simulink subsystem "PvtSubSys_LATC"  (R2020b)
settings: Solver=VariableStepAuto  StartTime=0.0  StopTime=10.0  RelTol=1e-3
values from neighbouring files (symbols this model uses):
  P_Global_CharSpd_ms : value not decoded    [PubParsGlobal.sldd]
  P_Global_SteeringAngleRatio : value not decoded    [PubParsGlobal.sldd]
  P_Global_WheelBase_m : value not decoded    [PubParsGlobal.sldd]
  P_LCS_A0_Limit = 0.25    [LATC.sldd]    (also in LCS_v05.sldd)
  P_LCS_A1_Limit = 0.002    [LATC.sldd]    (also in LCS_v05.sldd)
  P_LCS_communicationTest = 1.0    [LATC.sldd]    (also in LCS_v05.sldd)
  P_LCS_Current_Offset_Test_SW = 0.0    [LATC.sldd]
  P_LCS_Current_Offset_Test_Value = 0.0    [LATC.sldd]
  P_LCS_Curvature_bp : value not decoded    [LATC.sldd]
  P_LCS_CycleTime = 0.4 0.4 0.4 0.4 0.4 0.4 0.4 0.4 0.4 0.6 0.6 0.6 0.6 0.6 0.6 0.6 0.4 0.4 0.4 0.4 0.4 0.4 0.4 0.4 0.4 0.6 0.6 0.6 0.6 0.6 0.6 0.6 0.4 0.4 0.4 0.4 0.4 0.4 0.4 0.4 0.4 0.6 0.6 0.6 0.6 0.6 0.6 0.6 0.4 0.4 0.4 0.4 0.4 0.4 0.4 0.4 0.4 0.6 0.6 0.6 0.6 0.6 0.6 0.6 0.4 0.4 0.4 0.4 0.4 0.4 0.4 0.4 0.4 0.6 0.6 0.6 0.6 0.6 0.6 0.6 0.4 0.4 0.4 0.4 0.4 0.4 0.4 0.4 0.4 0.6 0.6 0.6 0.6 0.6 0.6 0.6 0.4 0.4 0.4 0.4    [LATC.sldd]
  P_LCS_ESS_AngleSlope_Limit = 2.9    [LATC.sldd]    (also in LCS_v05.sldd)
  P_LCS_IN_Offset_Test_SW = 0.0    [LATC.sldd]    (also in LCS_v05.sldd)
  P_LCS_IN_Offset_Test_Value = 0.0    [LATC.sldd]    (also in LCS_v05.sldd)
  P_LCS_LATC_CurOffsetVehicleSpdLimitValue_degs = 7.0    [LATC.sldd]
  P_LCS_LATC_Du_Max = 20.0    [LATC.sldd]
  P_LCS_LATC_ELKAngleSlope_ratio : value not decoded    [LATC.sldd]
  P_LCS_LATC_ELKMaxLatAcc_ms2 : value not decoded    [LATC.sldd]
  P_LCS_LATC_ESSAngleSlope_ratio : value not decoded    [LATC.sldd]
  P_LCS_LATC_ESSMaxLatAcc_ms2 : value not decoded    [LATC.sldd]
  P_LCS_LATC_LCAngleSlope_ratio : value not decoded    [LATC.sldd]
  P_LCS_LATC_LCCancleMaxLatAcc_ms2 : value not decoded    [LATC.sldd]
  P_LCS_LATC_LCEcoAngleSlope_ratio : value not decoded    [LATC.sldd]
  P_LCS_LATC_LCEcoMaxLatAcc_ms2 : value not decoded    [LATC.sldd]
  P_LCS_LATC_LCKAngleSlope_ratio : value not decoded    [LATC.sldd]
  P_LCS_LATC_LCKIEAngleSlope_ratio : value not decoded    [LATC.sldd]
  P_LCS_LATC_LCKIEMaxLatAcc_ms2 : value not decoded    [LATC.sldd]
  P_LCS_LATC_LCKMaxLatAcc_ms2 : value not decoded    [LATC.sldd]
  P_LCS_LATC_LCNormalAngleSlope_ratio : value not decoded    [LATC.sldd]
  P_LCS_LATC_LCNormalMaxLatAcc_ms2 : value not decoded    [LATC.sldd]
  P_LCS_LATC_LCSportAngleSlope_ratio : value not decoded    [LATC.sldd]
  P_LCS_LATC_LCSportMaxLatAcc_ms2 : value not decoded    [LATC.sldd]
  P_LCS_LATC_LKAAngleSlope_ratio : value not decoded    [LATC.sldd]
  P_LCS_LATC_LKAMaxLatAcc_ms2 : value not decoded    [LATC.sldd]
  P_LCS_LATC_MatrixQ1_st = 0.8 0.8 1.2 1.4 1.4 1.4 2.0 2.2 2.2 2.2 2.2 2.2 2.2 2.2 2.2 2.2 0.8 0.8 1.2 1.4 1.4 1.4 2.0 2.2 2.2 2.2 2.2 2.2 2.2 2.2 2.2 2.2 0.8 0.8 1.2 1.4 1.4 1.4 2.0 2.2 2.2 2.2 2.2 2.2 2.2 2.2 2.2 2.2 0.8 0.8 1.2 1.4 1.4 1.4 2.0 2.2 2.2 2.2 2.2 2.2 2.2 2.2 2.2 2.2 0.8 0.8 1.2 1.4 1.4 1.4 2.0 2.2 2.2 2.2 2.2 2.2 2.2 2.2 2.2 2.2 0.8 0.8 1.2 1.4 1.4 1.4 2.0 2.2 2.2 2.2 2.2 2.2 2.2 2.2 2.2 2.2 0.8 0.8 1.2 1.4    [LATC.sldd]
  P_LCS_LATC_MatrixQ3_st = 20.0 20.0 20.0 20.0 20.0 15.0 15.0 15.0 15.0 15.0 15.0 15.0 15.0 13.0 13.0 13.0 20.0 20.0 20.0 20.0 20.0 15.0 15.0 15.0 15.0 15.0 15.0 15.0 15.0 13.0 13.0 13.0 20.0 20.0 20.0 20.0 20.0 15.0 15.0 15.0 15.0 15.0 15.0 15.0 15.0 13.0 13.0 13.0 20.0 20.0 20.0 20.0 20.0 15.0 15.0 15.0 15.0 15.0 15.0 15.0 15.0 13.0 13.0 13.0 20.0 20.0 20.0 20.0 20.0 15.0 15.0 15.0 15.0 15.0 15.0 15.0 15.0 13.0 13.0 13.0    [LATC.sldd]
  P_LCS_LATC_MatrixR_st = 10.0 10.0 10.0 10.0 10.0 10.0 10.0 15.0 15.0 15.0 15.0 15.0 15.0 15.0 15.0 15.0 10.0 10.0 10.0 10.0 10.0 10.0 10.0 15.0 15.0 15.0 15.0 15.0 15.0 15.0 15.0 15.0 10.0 10.0 10.0 10.0 10.0 10.0 10.0 15.0 15.0 15.0 15.0 15.0 15.0 15.0 15.0 15.0 10.0 10.0 10.0 10.0 10.0 10.0 10.0 15.0 15.0 15.0 15.0 15.0 15.0 15.0 15.0 15.0 10.0 10.0 10.0 10.0 10.0 10.0 10.0 15.0 15.0 15.0 15.0 15.0 15.0 15.0 15.0 15.0    [LATC.sldd]
  P_LCS_LATC_Max_LatAcc = 4.0    [LATC.sldd]
  P_LCS_LATC_Max_Phi = 15.0    [LATC.sldd]
  P_LCS_LATC_Max_y = 0.5    [LATC.sldd]
  P_LCS_LATC_MPC_SW = 0.0    [LATC.sldd]
  P_LCS_LATC_PreView_SW = 1.0    [LATC.sldd]
  P_LCS_LATC_SoftConstWeight = 1.0    [LATC.sldd]
  P_LCS_LATC_StateActivAngleSlopeLimit_ratio : value not decoded    [LATC.sldd]
  P_LCS_LATC_StateActiveFlg_TabX_st : value not decoded    [LATC.sldd]
  P_LCS_LATC_StateActiveHoldTime_TabY_st : value not decoded    [LATC.sldd]
  P_LCS_LATC_StateHoldTime_st = 250.0    [LATC.sldd]
  P_LCS_LATC_TarAngleFliterWindowSize = 5.0    [LATC.sldd]
  P_LCS_LATC_TarAngleLP_Time = 0.02    [LATC.sldd]
  P_LCS_LATC_U_Max = 90.0    [LATC.sldd]
  P_LCS_LCK_AngleSlope_Limit = 1.4    [LATC.sldd]
  P_LCS_LineVaildSW = 0.0    [LATC.sldd]
  P_LCS_Lookahead_Distance : value not decoded    [LATC.sldd]
  P_LCS_Lookahead_DistanceFac : value not decoded    [LATC.sldd]
  P_LCS_PLAN_CurvePreView_s = 0.3    [LATC.sldd]
  P_LCS_PLAN_CurvePreview_TabX_m : value not decoded    [LATC.sldd]
  P_LCS_PLAN_CurvePreViewFilterTime_s = 0.1    [LATC.sldd]
  P_LCS_PLAN_ELKAyDtLimit_Tab_ms3 = 1.0 1.0 1.0 1.0 1.0 1.0 1.0 1.0 1.0 1.0 1.0 1.0 1.0 1.0 1.0 1.0 1.0 1.0 1.0 1.0 1.0 1.0 1.0 1.0 1.0 1.0 1.0 1.0 1.0 1.0 1.0 1.0 1.0 1.0 1.0 1.0 1.0 1.0 1.0 1.0 1.0 1.0 1.0 1.0 1.0 1.0 1.0 1.0 1.0 1.0 1.0 1.0 1.0 1.0 1.0 1.0 1.0 1.0 1.0 1.0 1.0 1.0 1.0 1.0 1.0 1.0 1.0 1.0 1.0 1.0 1.0 1.0 1.0 1.0 1.0 1.0 1.0 1.0 1.0 1.0 1.0 1.0 1.0 1.0 1.0 1.0 1.0 1.0 1.0 1.0 1.0 1.0 1.0 1.0 1.0 1.0 1.0 1.0 1.0 1.0    [LATC.sldd]
  P_LCS_PLAN_ESSAyDtLimit_Tab_ms3 = 1.0 1.0 1.0 1.0 1.0 1.0 1.0 1.0 1.0 1.0 1.0 1.0 1.0 1.0 1.0 1.0 1.0 1.0 1.0 1.0 1.0 1.0 1.0 1.0 1.0 1.0 1.0 1.0 1.0 1.0 1.0 1.0 1.0 1.0 1.0 1.0 1.0 1.0 1.0 1.0 1.0 1.0 1.0 1.0 1.0 1.0 1.0 1.0 1.0 1.0 1.0 1.0 1.0 1.0 1.0 1.0 1.0 1.0 1.0 1.0 1.0 1.0 1.0 1.0 1.0 1.0 1.0 1.0 1.0 1.0 1.0 1.0 1.0 1.0 1.0 1.0 1.0 1.0 1.0 1.0 1.0 1.0 1.0 1.0 1.0 1.0 1.0 1.0 1.0 1.0 1.0 1.0 1.0 1.0 1.0 1.0 1.0 1.0 1.0 1.0    [LATC.sldd]
  P_LCS_PLAN_LCCancleAyDtLimit_Tab_ms3 = 1.0 1.0 1.0 1.0 1.0 1.0 1.0 1.0 1.0 1.0 1.0 1.0 1.0 1.0 1.0 1.0 1.0 1.0 1.0 1.0 1.0 1.0 1.0 1.0 1.0 1.0 1.0 1.0 1.0 1.0 1.0 1.0 1.0 1.0 1.0 1.0 1.0 1.0 1.0 1.0 1.0 1.0 1.0 1.0 1.0 1.0 1.0 1.0 1.0 1.0 1.0 1.0 1.0 1.0 1.0 1.0 1.0 1.0 1.0 1.0 1.0 1.0 1.0 1.0 1.0 1.0 1.0 1.0 1.0 1.0 1.0 1.0 1.0 1.0 1.0 1.0 1.0 1.0 1.0 1.0 1.0 1.0 1.0 1.0 1.0 1.0 1.0 1.0 1.0 1.0 1.0 1.0 1.0 1.0 1.0 1.0 1.0 1.0 1.0 1.0    [LATC.sldd]
  P_LCS_PLAN_LCEcoAyDtLimit_Tab_ms3 = 1.0 1.0 1.0 1.0 1.0 1.0 1.0 1.0 1.0 1.0 1.0 1.0 1.0 1.0 1.0 1.0 1.0 1.0 1.0 1.0 1.0 1.0 1.0 1.0 1.0 1.0 1.0 1.0 1.0 1.0 1.0 1.0 1.0 1.0 1.0 1.0 1.0 1.0 1.0 1.0 1.0 1.0 1.0 1.0 1.0 1.0 1.0 1.0 1.0 1.0 1.0 1.0 1.0 1.0 1.0 1.0 1.0 1.0 1.0 1.0 1.0 1.0 1.0 1.0 1.0 1.0 1.0 1.0 1.0 1.0 1.0 1.0 1.0 1.0 1.0 1.0 1.0 1.0 1.0 1.0 1.0 1.0 1.0 1.0 1.0 1.0 1.0 1.0 1.0 1.0 1.0 1.0 1.0 1.0 1.0 1.0 1.0 1.0 1.0 1.0    [LATC.sldd]
  P_LCS_PLAN_LCKAyDtLimit_Tab_ms3 = 1.5 1.5 1.5 1.5 1.5 1.5 1.5 1.5 1.5 1.5 1.5 1.5 1.5 1.5 1.5 1.5 1.5 1.5 1.5 1.5 1.5 1.5 1.5 1.5 1.5 1.5 1.5 1.5 1.5 1.5 1.5 1.5 1.5 1.5 1.5 1.5 1.5 1.5 1.5 1.5 1.5 1.5 1.5 1.5 1.5 1.5 1.5 1.5 1.5 1.5 1.5 1.5 1.5 1.5 1.5 1.5 1.5 1.5 1.5 1.5 1.5 1.5 1.5 1.5 1.5 1.5 1.5 1.5 1.5 1.5 1.5 1.5 1.5 1.5 1.5 1.5 1.5 1.5 1.5 1.5 1.5 1.5 1.5 1.5 1.5 1.5 1.5 1.5 1.5 1.5 1.5 1.5 1.5 1.5 1.5 1.5 1.5 1.5 1.5 1.5    [LATC.sldd]
  P_LCS_PLAN_LCKIEAyDtLimit_Tab_ms3 = 1.0 1.0 1.0 1.0 1.0 1.0 1.0 1.0 1.0 1.0 1.0 1.0 1.0 1.0 1.0 1.0 1.0 1.0 1.0 1.0 1.0 1.0 1.0 1.0 1.0 1.0 1.0 1.0 1.0 1.0 1.0 1.0 1.0 1.0 1.0 1.0 1.0 1.0 1.0 1.0 1.0 1.0 1.0 1.0 1.0 1.0 1.0 1.0 1.0 1.0 1.0 1.0 1.0 1.0 1.0 1.0 1.0 1.0 1.0 1.0 1.0 1.0 1.0 1.0 1.0 1.0 1.0 1.0 1.0 1.0 1.0 1.0 1.0 1.0 1.0 1.0 1.0 1.0 1.0 1.0 1.0 1.0 1.0 1.0 1.0 1.0 1.0 1.0 1.0 1.0 1.0 1.0 1.0 1.0 1.0 1.0 1.0 1.0 1.0 1.0    [LATC.sldd]
  P_LCS_PLAN_LCNormalAyDtLimit_Tab_ms3 = 1.0 1.0 1.0 1.0 1.0 1.0 1.0 1.0 1.0 1.0 1.0 1.0 1.0 1.0 1.0 1.0 1.0 1.0 1.0 1.0 1.0 1.0 1.0 1.0 1.0 1.0 1.0 1.0 1.0 1.0 1.0 1.0 1.0 1.0 1.0 1.0 1.0 1.0 1.0 1.0 1.0 1.0 1.0 1.0 1.0 1.0 1.0 1.0 1.0 1.0 1.0 1.0 1.0 1.0 1.0 1.0 1.0 1.0 1.0 1.0 1.0 1.0 1.0 1.0 1.0 1.0 1.0 1.0 1.0 1.0 1.0 1.0 1.0 1.0 1.0 1.0 1.0 1.0 1.0 1.0 1.0 1.0 1.0 1.0 1.0 1.0 1.0 1.0 1.0 1.0 1.0 1.0 1.0 1.0 1.0 1.0 1.0 1.0 1.0 1.0    [LATC.sldd]
  P_LCS_PLAN_LCSportAyDtLimit_Tab_ms3 = 1.0 1.0 1.0 1.0 1.0 1.0 1.0 1.0 1.0 1.0 1.0 1.0 1.0 1.0 1.0 1.0 1.0 1.0 1.0 1.0 1.0 1.0 1.0 1.0 1.0 1.0 1.0 1.0 1.0 1.0 1.0 1.0 1.0 1.0 1.0 1.0 1.0 1.0 1.0 1.0 1.0 1.0 1.0 1.0 1.0 1.0 1.0 1.0 1.0 1.0 1.0 1.0 1.0 1.0 1.0 1.0 1.0 1.0 1.0 1.0 1.0 1.0 1.0 1.0 1.0 1.0 1.0 1.0 1.0 1.0 1.0 1.0 1.0 1.0 1.0 1.0 1.0 1.0 1.0 1.0 1.0 1.0 1.0 1.0 1.0 1.0 1.0 1.0 1.0 1.0 1.0 1.0 1.0 1.0 1.0 1.0 1.0 1.0 1.0 1.0    [LATC.sldd]
  P_LCS_PLAN_LKAAyDtLimit_Tab_ms3 = 1.0 1.0 1.0 1.0 1.0 1.0 1.0 1.0 1.0 1.0 1.0 1.0 1.0 1.0 1.0 1.0 1.0 1.0 1.0 1.0 1.0 1.0 1.0 1.0 1.0 1.0 1.0 1.0 1.0 1.0 1.0 1.0 1.0 1.0 1.0 1.0 1.0 1.0 1.0 1.0 1.0 1.0 1.0 1.0 1.0 1.0 1.0 1.0 1.0 1.0 1.0 1.0 1.0 1.0 1.0 1.0 1.0 1.0 1.0 1.0 1.0 1.0 1.0 1.0 1.0 1.0 1.0 1.0 1.0 1.0 1.0 1.0 1.0 1.0 1.0 1.0 1.0 1.0 1.0 1.0 1.0 1.0 1.0 1.0 1.0 1.0 1.0 1.0 1.0 1.0 1.0 1.0 1.0 1.0 1.0 1.0 1.0 1.0 1.0 1.0    [LATC.sldd]
  P_LCS_PLAN_MinPlanDis_m : value not decoded    [LATC.sldd]
  P_LCS_PLAN_PreCurMinDisFac_ratio : value not decoded    [LATC.sldd]
  P_LCS_PLAN_PreDisCurve_TabX_m : value not decoded    [LATC.sldd]
  P_LCS_PLAN_StateActiv_AyDtLimit_ms3 : value not decoded    [LATC.sldd]
  P_LCS_PLAN_VehicleSpd_TabX_kph : value not decoded    [LATC.sldd]
  P_LCS_PLAN_VehicleSpd_TabY_Kph : value not decoded    [LATC.sldd]
  P_LCS_Trq_Switch = 0.0    [LATC.sldd]    (also in LCS_v05.sldd)
  P_LCS_VehicleSpd_TabX_Kph : value not decoded    [LATC.sldd]
undefined symbols (not defined in the file or in its folder): HWP_AngCmdReqVal, HWP_AngCmdReqValVld, HWP_FuncTrqCmdReqFlag, HWP_ReqCtrlEPS, HWP_ReqCtrlEPSVld, HWP_TrqOvlCmdReqValue, HWP_WorkReq, HWP_WorkReqVld
libraries: simulink x4, dspbuff3 x2
(part 7 of 8)

== matlab function PvtSubSys_LATC/LATC/LateralControl/LCS_Angle/Controller/StateErrorCalc/MATLAB Function2 ==
  data: Ego_X input; Ego_Y input; Ego_Heading input; Ego_Spd input; Ego_Acc input; Ego_YawRate input; lookahead_Pt_X input; lookahead_Pt_Y input; lookahead_Pt_Heading input; lookahead_Pt_Kappa input; Project_Pt_X input; Project_Pt_Y input; Project_Pt_Heading input; Project_Pt_Kappa input; lat_error output; lat_error_rate output; heading_error output; heading_error_rate output; lat_error_lookahead output; lat_error_rate_lookahead output; heading_error_lookahead output; heading_error_rate_lookahead output
function [lat_error,lat_error_rate,heading_error,heading_error_rate,lat_error_lookahead,lat_error_rate_lookahead,heading_error_lookahead,heading_error_rate_lookahead] ...
          = ComputeLatErrors(Ego_X,Ego_Y,Ego_Heading,Ego_Spd,Ego_Acc,Ego_YawRate,lookahead_Pt_X,lookahead_Pt_Y,lookahead_Pt_Heading,lookahead_Pt_Kappa,Project_Pt_X,Project_Pt_Y,Project_Pt_Heading,Project_Pt_Kappa)
    %% 横向控制中的误差计算  
    % 感觉存在问题，打算计算两套误差状态，一个是基于车辆与垂直点的误差，一个是车辆与预瞄点的误差。再加上前边车辆的位置推算模块
    
    % 角度误差计算
    curr_heading = Ego_Heading;
    heading_error = curr_heading-Project_Pt_Heading; % 车辆朝向角与垂直点朝向角误差
    heading_error = NormalizeAngle(heading_error);
    heading_error_lookahead = curr_heading-lookahead_Pt_Heading; % 车辆朝向角与预瞄点朝向误差
    heading_error_lookahead = NormalizeAngle(heading_error_lookahead);
    % 垂直点偏差计算
    X_curr = Ego_X;
    Y_curr = Ego_Y;
    dx = X_curr - Project_Pt_X;
    dy = Y_curr - Project_Pt_Y;
    lat_error = cos(Project_Pt_Heading)*dy-sin(Project_Pt_Heading)*dx;
    lat_error_rate=Ego_Spd*sin(heading_error);
    Project_Pt_YawRate = Project_Pt_Kappa*Ego_Acc;
    heading_error_rate = Ego_YawRate-Project_Pt_YawRate;
    % 预瞄点的偏差计算
    dx_pre = X_curr - lookahead_Pt_X;
    dy_pre = Y_curr - lookahead_Pt_Y;
    lat_error_lookahead = cos(lookahead_Pt_Heading)*dy_pre-sin(lookahead_Pt_Heading)*dx_pre;
    lat_error_rate_lookahead=Ego_Spd*sin(heading_error_lookahead);
    lookahead_Pt_YawRate = lookahead_Pt_Kappa*Ego_Acc;
    heading_error_rate_lookahead = Ego_YawRate-lookahead_Pt_YawRate;
end
function res_angle=NormalizeAngle(origin_angle)
%% 角度规范化，heading角在-pi~pi之间
    res_angle=mod(origin_angle+pi,2*pi);
    if (res_angle<0)
        res_angle=res_angle+2*pi;
    end
    res_angle=res_angle-pi;
end

% tor=[cos(thetar);sin(thetar)];
% nor=[-sin(thetar);cos(thetar)];
% d_err=[x-xr;y-yr];
% ed=nor'*d_err;
% es=tor'*d_err;
% %projection_point_thetar=thetar(dmin);%apollo
% projection_point_thetar=thetar+kappar*es;
% ed_dot=vy*cos(phi-projection_point_thetar)+vx*sin(phi-projection_point_thetar);
% %%%%%%%%%
% ephi=sin(phi-projection_point_thetar);
% %%%%%%%%%
% ss_dot=vx*cos(phi-projection_point_thetar)-vy*sin(phi-projection_point_thetar);
% s_dot=ss_dot/(1-kappar*ed);
% ephi_dot=phi_dot-kappar*s_dot;

== matlab function PvtSubSys_LATC/LATC/LateralControl/LCS_Angle/Controller/StateErrorCalc/Reference_Point_Select/MatchPoint_ProjectPoint ==
  data: CurPosX input; CurPosY input; MatchPtX output; MatchPtY output; MatchPtTheta output; MatchPtCurve output; MatchPtS output; RefTrajX input; ProjectPtX output; ProjectPtY output; RefTrajY input; RefTrajTheta input; RefTrajCurve input; ProjectPtTheta output; ProjectPtCurve output; RefTrajS input; ProjectPtS output
function [MatchPtX,MatchPtY,MatchPtTheta,MatchPtCurve,MatchPtS,ProjectPtX,ProjectPtY,ProjectPtTheta,ProjectPtCurve,ProjectPtS] ...
           = SearchProjectPoint(CurPosX,CurPosY,RefTrajX,RefTrajY,RefTrajTheta,RefTrajCurve,RefTrajS)
PathPtNum = single(length(RefTrajX));
Index = single(0);
MinDis = single(10000);
% 声明increase_count，用于表示在遍历时distance连续增加的个数
increase_count = 0;

for i = 1:PathPtNum
    Dis = sqrt((CurPosX-RefTrajX(i,1))*(CurPosX-RefTrajX(i,1))+(CurPosY-RefTrajY(i,1))*(CurPosY-RefTrajY(i,1)));
    if (Dis < MinDis)
        MinDis = Dis;
        Index = i;
        increase_count = 0;
    else
        increase_count = increase_count + 1;
    end
    %如果distance连续增加20次就不要再遍历了，节省时间
    if increase_count > 20
        break;
    end
end
% 找到匹配点索引MatchPoint
MatchPtX = RefTrajX(Index,1);
MatchPtY = RefTrajY(Index,1);
MatchPtTheta = RefTrajTheta(Index,1);
MatchPtCurve = RefTrajCurve(Index,1);
MatchPtS = RefTrajS(Index,1);
%求解垂直点坐标ProjectPoint
if (Index == 1) %第一个点
    PointEgoX = CurPosX;
    PointEgoY = CurPosY;
    PointA_X = RefTrajX(1,1);
    PointA_Y = RefTrajY(1,1);
    PointB_X = RefTrajX(2,1);
    PointB_Y = RefTrajY(2,1);
    DotProductA = DotProduct(PointA_X,PointA_Y,PointEgoX,PointEgoY,PointB_X,PointB_Y);
    DotProductB = DotProduct(PointB_X,PointB_Y,PointEgoX,PointEgoY,PointA_X,PointA_Y);
    if(DotProductA>=0 && DotProductB>=0)
        IndexA = single(1);
        IndexB = single(2);
    else
        IndexA = single(1);
        IndexB = single(1);
    end
elseif (Index == PathPtNum)%最后一个点
    PointEgoX = CurPosX;
    PointEgoY = CurPosY;
    PointA_X = RefTrajX(PathPtNum-1,1);
    PointA_Y = RefTrajY(PathPtNum-1,1);
    PointB_X = RefTrajX(PathPtNum,1);
    PointB_Y = RefTrajY(PathPtNum,1);
    DotProductA = DotProduct(PointA_X,PointA_Y,PointEgoX,PointEgoY,PointB_X,PointB_Y);
    DotProductB = DotProduct(PointB_X,PointB_Y,PointEgoX,PointEgoY,PointA_X,PointA_Y);
    if(DotProductA>=0 && DotProductB>=0)
        IndexA = PathPtNum-1;
        IndexB = PathPtNum;
    else
        IndexA = PathPtNum;
        IndexB = PathPtNum;
    end
else
    PointEgoX = CurPosX;
    PointEgoY = CurPosY;
    PointA_X = RefTrajX(Index,1);
    PointA_Y = RefTrajY(Index,1);
    PointB_X = RefTrajX(Index+1,1);
    PointB_Y = RefTrajY(Index+1,1);
    DotProductA = DotProduct(PointA_X,PointA_Y,PointEgoX,PointEgoY,PointB_X,PointB_Y);
    DotProductB = DotProduct(PointB_X,PointB_Y,PointEgoX,PointEgoY,PointA_X,PointA_Y);
    if(DotProductA>=0 && DotProductB>=0)
        IndexA = Index;
        IndexB = Index+1;
    else
        IndexA = Index;
        IndexB = Index-1;
    end
end
% 投影点坐标求解
PointA_X = RefTrajX(IndexA,1);
PointA_Y = RefTrajY(IndexA,1);
PointB_X = RefTrajX(IndexB,1);
PointB_Y = RefTrajY(IndexB,1);
[ProjectPtX,ProjectPtY] = Pt2LineProject(PointEgoX,PointEgoY,PointA_X,PointA_Y,PointB_X,PointB_Y);
% 求解投影点的朝向角和曲率
LengthOA = CalTwoPtLength(ProjectPtX,ProjectPtY,PointA_X,PointA_Y);
LengthAB = CalTwoPtLength(PointA_X,PointA_Y,PointB_X,PointB_Y);
if ( LengthAB < 0.001)
    fWeight = single(1);
else
    fWeight = single(LengthOA/LengthAB);
end
ProjectPtTheta = RefTrajTheta(IndexA,1)*fWeight + RefTrajTheta(IndexB,1)*(1-fWeight);
ProjectPtCurve = RefTrajCurve(IndexA,1)*fWeight + RefTrajCurve(IndexB,1)*(1-fWeight);
if IndexA > IndexB
    ProjectPtS =  RefTrajS(IndexA,1) - LengthAB*fWeight;
elseif IndexA < IndexB
    ProjectPtS =  RefTrajS(IndexA,1) + LengthAB*fWeight;
else
    ProjectPtS =  RefTrajS(IndexA,1);
end
end

function DotProduct_Result = DotProduct(X1,Y1,X2,Y2,X3,Y3)
DotProduct_Result = (X2 - X1)*(X3 - X1) + (Y2 - Y1)*(Y3 - Y1);
end
function [ProjectPtX,ProjectPtY] = Pt2LineProject(X,Y,X1,Y1,X2,Y2)
%X = single(0);Y = single(0);X1 = single(0);Y1 = single(0);X2 = single(0);Y2 = single(0);
if (abs((X2-X1)*(X2-X1) + (Y2-Y1)*(Y2-Y1)) > 0.0001)
    ProjectPtX = (X*(X2-X1)*(X2-X1)+Y*(Y2-Y1)*(X2-X1)+(X1*Y2-X2*Y1)*(Y2-Y1))/((X2-X1)*(X2-X1)+(Y2-Y1)*(Y2-Y1));
    ProjectPtY = (X*(X2-X1)*(Y2-Y1)+Y*(Y2-Y1)*(Y2-Y1)+(X2*Y1-X1*Y2)*(X2-X1))/((X2-X1)*(X2-X1)+(Y2-Y1)*(Y2-Y1));
else
    ProjectPtX = X1;
    ProjectPtY = Y1;
end
end
function Length = CalTwoPtLength(X1,Y1,X2,Y2)
Length = sqrt((X1-X2)*(X1-X2) + (Y1-Y2)*(Y1-Y2));
end

== matlab function PvtSubSys_LATC/LATC/LateralControl/LCS_Angle/Controller/StateErrorCalc/Reference_Point_Select/MATLAB Function1 ==
  data: Pt1X input; Dis output; Pt1Y input; Pt2X input; Pt2Y input; AbsDis output
function [Dis,AbsDis]= fcn(Pt1X,Pt1Y,Pt2X,Pt2Y)
Dis = (sqrt((Pt1X-Pt2X)*(Pt1X-Pt2X)+(Pt1Y-Pt2Y)*(Pt1Y-Pt2Y)))*sign(Pt1Y);
AbsDis = sqrt((Pt1X-Pt2X)*(Pt1X-Pt2X)+(Pt1Y-Pt2Y)*(Pt1Y-Pt2Y));
end

== matlab function PvtSubSys_LATC/LATC/LateralControl/LCS_Angle/Controller/StateErrorCalc/Reference_Point_Select/MATLAB Function2 ==
  data: path_x output; path_y output; path_x input; path_heading output; path_y input; path_kappa output; path_s output
function [path_x,path_y,path_heading,path_kappa,path_s] = fcn(path_x,path_y)
%该模块是直接采用的老王模型中的通用模块
%该函数将计算path的切线方向与x轴的夹角和曲率
%输入：path_x,y路径坐标
%输出：path heading kappa 路径的heading和曲率
%原理 heading = arctan(dy/dx);
%     kappa = dheading/ds;
%     ds = (dx^2 + dy^2)^0.5

%注意，角度的多值性会带来很大的麻烦，需要慎重处理
%例，x 与 x + 2pi往往代表同一个角度，这种多值性在计算曲率会带来麻烦
%比如 原本是(0.1 - (-0.1))/ds，但如果计算出的-0.1多了一个2pi
%kappa就等于(0.1 - (-0.1 + 2*pi))/ds，曲率会变得非常大
%还有若采用中点欧拉法计算heading时，(即使用(y2 - y1)/(x2 - x1)的反正切计算一个角度 ，用(y1 - y0)/(x1
%-x0)的反正切又计算一个角度，然后加起来除以2),如果精确值是 (a1 + a2)/2,但最终计算的结果可能是(a1 + a2 + 2pi)/2
% 还有 tan(x) = tan(x + pi) 所以arctan(tan(x))可能等于x，也可能等于x + pi
% 角度的处理非常麻烦，而且角度处理不当往往是许多奇怪错误的源头

dx = diff(path_x);
dy = diff(path_y);
%用中点欧拉法要比向前欧拉法向后欧拉法更精确，但是也可能计算出的结果比精确值多一个pi
%在这里对dx,dy做中点欧拉法，使用四象限反正切计算角度
dx_pre = [dx(1);dx];
dx_after = [dx;dx(end)];
dx_final = (dx_pre + dx_after)/2;

dy_pre = [dy(1);dy];
dy_after = [dy;dy(end)];
dy_final = (dy_pre + dy_after)/2;

ds_final = sqrt(dx_final.^2 + dy_final.^2);
cum_ds = cumsum(ds_final);
path_heading = atan2(dy_final,dx_final);

dheading = diff(path_heading);
dheading_pre = [dheading(1);dheading];
dheading_after = [dheading;dheading(end)];
dheading_final = (dheading_pre + dheading_after) / 2;
%为了防止dheading出现多一个2pi的错误，假设真实的dheading较小，用sin(dheading)近似dheading
path_kappa = sin(dheading_final) ./ ds_final;
path_s = single(zeros(length(path_x),1));
path_s(2:end,1) = cum_ds(1:end-1,1);
end

== matlab function PvtSubSys_LATC/LATC/LateralControl/LCS_Angle/Controller/StateErrorCalc/EgoMovement ==
  data: dDeltaX output single size=1; dDeltaY output single size=1; tCycle input single size=1; CosOfPsi output single size=1; Kap input single size=1; psiDtOptSync input single size=1; Vego input single size=1; alpSideSlipAngle input single size=1; SinOfPsi output single size=1; ego_x input; ego_y input; ego_heading input; predict_x output; predict_y output; predict_heading output; predict_spd output; predict_yawrate output
function [dDeltaX,dDeltaY,CosOfPsi,SinOfPsi,predict_x,predict_y,predict_heading,predict_spd,predict_yawrate] = EgoVehicleMovement(tCycle,Kap,psiDtOptSync,Vego,alpSideSlipAngle,ego_x,ego_y,ego_heading)
%#codegen
if Kap==0
    dDeltaX = Vego*tCycle;
    dDeltaY = single(0);
    CosOfPsi = single(1);
    SinOfPsi = single(0);
    t_Psi = single(0);
else
    t_kap = Kap;
    if ((Kap>0.125)||(Kap<-0.125))&&(Vego>1)
        t_kapPsiDtSync = psiDtOptSync/Vego;    %实际计算的曲率
        if abs(t_kapPsiDtSync)>abs(Kap)          
            t_kap = t_kapPsiDtSync;
        end
    end
    t_Psi = t_kap*Vego*tCycle;
    SinOfPsi = sin(t_Psi);
    CosOfPsi = cos(t_Psi);
    t_dDeltaXTemp = SinOfPsi/t_kap;
    t_dDeltaYTemp = 2*(sin(t_Psi/2)*sin(t_Psi/2))/t_kap;
    dDeltaX = cos(alpSideSlipAngle)*t_dDeltaXTemp - sin(alpSideSlipAngle)*t_dDeltaYTemp;
    dDeltaY = sin(alpSideSlipAngle)*t_dDeltaXTemp + cos(alpSideSlipAngle)*t_dDeltaYTemp;
end
predict_x = ego_x + dDeltaX;
predict_y = ego_y + dDeltaY;
predict_heading = ego_heading + t_Psi;
predict_spd = Vego;
predict_yawrate = psiDtOptSync;
end

== matlab function PvtSubSys_LATC/LATC/LateralControl/LCS_Angle/Controller/TargetAngleCalc/MATLAB Function1 ==
  data: ControlValid input; Final_steer_angle_cmd output; SteerAngle input; CurrentSteerAngleOffset input; Veh_Speed input; ref_curvature input; lateral_error input; lateral_error_rate input; heading_error input; heading_error_rate input; Left_steer_ratio input; Right_steer_ratio input; Matrix_q1 input; Matrix_q3 input; Matrix_R input; U_Max input; Du_Max input; LatError_contribution output; LatErrorRate_contribution output; HeadingError_contribution output; HeadingErrorRate_contribution output; steer_angle_cmd output; SoftConstWeight input
function [Final_steer_angle_cmd,LatError_contribution,LatErrorRate_contribution,...
    HeadingError_contribution,HeadingErrorRate_contribution,steer_angle_cmd]= ...
    MPC_Error_Du_Algorithm(ControlValid,SteerAngle,CurrentSteerAngleOffset,Veh_Speed,ref_curvature,lateral_error,lateral_error_rate,heading_error,heading_error_rate,...
    Left_steer_ratio,Right_steer_ratio,Matrix_q1,Matrix_q3,Matrix_R,U_Max,Du_Max,SoftConstWeight)

LatError_contribution = single(0);
LatErrorRate_contribution = single(0);
HeadingError_contribution = single(0);
HeadingErrorRate_contribution = single(0);
if ControlValid
    %% 1.车辆参数
    %1.1 车的大小及长度参数
    veh_params.vehicle_length = single(4.875);
    veh_params.vehicle_width  = single(2.2);
    veh_params.vehicle_height = single(1.69);
    %1.2 车辆控制参数
    veh_params.wheel_base = single(2.92);               %轴距, m
    veh_params.Vch = single(23.5);                      %特征车速
    veh_params.mu = single(1.0);                        %路面摩擦限制
    veh_params.max_acceleration = single(2);            %车辆最大加速度
    veh_params.max_deceleration = single(-2);           %车辆最大减速度
    veh_params.left_steer_ratio = Left_steer_ratio;     %车辆左侧转向传动比%
    veh_params.right_steer_ratio = Right_steer_ratio;   %车辆右侧转向传动比%
    veh_params.cf = single(2*55000);                    %车辆前轮侧偏刚度N/rad(两侧轮胎等效为一个*2)
    veh_params.cr = single(2*75000);                    %车辆后轮侧偏刚度N/rad
    veh_params.mass_fl = single(520);                   %车辆左前轮负重
    veh_params.mass_fr = single(520);                   %车辆右前轮负重
    veh_params.mass_rl = single(520);                   %车辆左后轮负重
    veh_params.mass_rr = single(520);                   %车辆右后轮负重
    %1.3 方向盘转角转换为车轮转角+度转弧度
    if (SteerAngle>=single(0))
        steer_transmission_ratio = veh_params.left_steer_ratio;
    else
        steer_transmission_ratio = veh_params.right_steer_ratio;
    end
    FrontWheel_AngleK1_rad = SteerAngle / (single(57.3) * steer_transmission_ratio);%反算前轮转角并转换成弧度制
    %% 2.控制参数计算
    mass_front =  veh_params.mass_fl + veh_params.mass_fr;
    mass_rear  =  veh_params.mass_rl + veh_params.mass_rr;
    mass =  mass_front + mass_rear;
    % lf = veh_params.wheel_base * (single(1.0) - mass_front / mass);% distance from front tires to cg, m
    % lr = veh_params.wheel_base * (single(1.0) - mass_rear / mass);% distance from rear tires to cg, m
    lf = single(1.27);% distance from front tires to cg,实际测试结果
    lr = single(1.64);% distance from rear tires to cg, m 实际测试结果
    iz = lf * lf * mass_front + lr * lr * mass_rear;
    %---------------------------求车辆响应增益---------------------------%
    % % 车辆模型，状态为[beta,wr]
    % 求车辆响应增益
    Veh_Speed = (max(Veh_Speed, single(0.2)));
    AAr = [(veh_params.cf+veh_params.cr),((veh_params.cf*lf-veh_params.cr*lr)/Veh_Speed)+mass*Veh_Speed;
           (veh_params.cf*lf-veh_params.cr*lr),(veh_params.cf*lf^2+veh_params.cr*lr^2)/Veh_Speed];
    BBr = [veh_params.cf;veh_params.cf*lf];
    a11 = AAr(1,1);
    a12 = AAr(1,2);
    a21 = AAr(2,1);
    a22 = AAr(2,2);
    b1 = BBr(1);
    b2 = BBr(2);
    %Ta = a11+a22;
    Da = a11*a22-a12*a21;
    
    Gr = (b2.*a11-b1.*a21)./Da; % 稳态横摆角速度增益，理想化增益是偏大，因为轮胎侧偏刚度会变小
    % Gb = (b1.*a22-b2.*a12)./Da; % 稳态质心侧偏角增益，理想化增益是偏大，因为轮胎侧偏刚度会变小
    Gay = Gr*Veh_Speed; % 稳态侧向加速度增益，理想化增益是偏大，因为轮胎侧偏刚度会变小
    %% 3.mpc算法
    % % 基于偏差的状态方程
    A=[0,1,0,0;
       0,-(veh_params.cf+veh_params.cr)/mass/Veh_Speed,(veh_params.cf+veh_params.cr)/mass,(-veh_params.cf*lf+veh_params.cr*lr)/mass/Veh_Speed;
       0,0,0,1;
       0,-(veh_params.cf*lf-veh_params.cr*lr)/iz/Veh_Speed,(veh_params.cf*lf-veh_params.cr*lr)/iz,-(veh_params.cf*lf^2+veh_params.cr*lr^2)/iz/Veh_Speed];
    B=[0;veh_params.cf/mass;0;veh_params.cf*lf/iz];
    C=[0;-(veh_params.cf*lf-veh_params.cr*lr)/mass/Veh_Speed-Veh_Speed;0;-(veh_params.cf*lf^2+veh_params.cr*lr^2)/iz/Veh_Speed];
    %-----------------------------------------------------------------%
    Q = single(zeros(4,4));
    Q(1,1) = Matrix_q1;                      %调整q矩阵的第一、三个参数，改善转向性能0.0001,0.02  Q为状态权重系数
    Q(3,3) = Matrix_q3;
    % R = single(zeros(1,1));
    R = Matrix_R;                            %R为控制量权重系数 R=1
    %-------------------状态方程离散化----------------------------------%
    Ts = single(0.02);
    Ad = single((eye(4)+A*Ts/2)/(eye(4)-A*Ts/2));
    Bd = single(Ts*B);
    Cd = single(Ts*C);
    %----------------扩展状态矩阵，将输入由绝对量变为增量----------------%
    Nu = 1;% 控制维数
    Nx = 4;% 原状态维数
    Ae = [Ad,Bd;zeros(Nu,Nx),eye(Nu)];%5*5
    Be = [Bd;eye(Nu)];%5*1
    Ce = [Cd;zeros(Nu)];%5*1
    Qe = [Q,zeros(Nx,Nu);zeros(Nu,Nx),R];%不能是1，应该是R,主要是考虑方向盘角度大小的矩阵大小
    Re = R; %1*1
    % % MPC预测模型
    Np = single(10); %预测步长
    Nc = single(3); % 控制步长
    [Ae_row,Ae_col] = size(Ae);%5*5
    [Be_row,Be_col] = size(Be);%5*1
    [Qe_row,Qe_col] = size(Qe);%5*1
    [Re_row,Re_col] = size(Re);%5*5
    [Ce_row,Ce_col] = size(Ce);%5*1
    At = single(zeros(Np*Ae_row,Ae_col));% 25*5
    Bt_c = single(zeros(Np*Ae_row,Np*Be_col)); % 25*25
    Bt_c_temp = single(zeros(Ae_row,Np*Be_col));% 5*25
    Qt = single(zeros(Np*Qe_row,Np*Qe_col)); % 25*25
    Ct = single(zeros(Np*Ce_row,Ce_col));% 25*1
    Ct_temp = single(zeros(Ce_row,Ce_col));% 5*1
    for r = 1:Np
        for c=1:Np
            if c<=r
                Bt_c_temp(:,((c-1)*Nu+1):c*Nu) = Ae^(r-c)*Be;%5*1
            end
            if c==r
                Qt(((r-1)*Qe_row)+1:r*Qe_row,((r-1)*Qe_col)+1:r*Qe_col) = Qe;% 25*25
            end
        end
        At(((r-1)*Ae_row+1):r*Ae_row,:) = Ae^r;
        Bt_c(((r-1)*Be_row+1):r*Be_row,:) = Bt_c_temp;
        Ct_temp = Ct_temp + Ae^(r-1)*Ce;
        Ct(((r-1)*Ce_row+1):r*Ce_row,:) = Ct_temp;
    end
    Rt = single(zeros(Nc*Re_row,Nc*Re_col));% 25*25
    for i = 1:Nc
        for j = 1:Nc
            if i==j
                Rt(((i-1)*Re_row)+1:i*Re_row,((i-1)*Re_col)+1:i*Re_col) = Re;
            end
        end
    end
    Bt = Bt_c(:,1:Nc); % 25*25
    %--------------------------约束矩阵生成--------------------------------%
    % 不等式约束,方向盘转角绝对值上下限
    A_k = zeros(Nc,Nc);%5*5
    for p=1:Nc
        for q=1:Nc
            if q<=p
                A_k(p,q)=1;
            else
                A_k(p,q)=0;
            end
        end
    end
    A_I = kron(A_k,eye(Nu));%求克罗内克积 5*5
    A_cons0 = [A_I,zeros(Nu*Nc,1); -A_I,zeros(Nu*Nc,1)]; % 后边增加一列0，主要是因为控制增量最后加了一个松弛因子，这里加一列0与松弛因子相乘，排除松弛因子的影响。10*6
    Delta_max = U_Max/single(57.3); % 车轮转角限制，由最大方向盘转角转换为车轮最大转角并转换成rad
    Delta_Max = kron(ones(Nc,1),Delta_max); % 5*1
    b_cons_coeff0 = [Delta_Max;Delta_Max]; % 10*1
    
    % % 增加软约束，为了舒适性，希望侧向加速度<4m/s^2，否则增加惩罚
    Ay_softbound = 4;% 为了舒适性，希望侧向加速度<4m/s^2，否则增加惩罚
    Ay_SoftBound=kron(ones(Nc,1),Ay_softbound); % 5*1
    A_cons1=[Gay*eye(Nu*Nc)*A_I,-ones(Nu*Nc,1);-Gay*eye(Nu*Nc)*A_I,-ones(Nu*Nc,1)];% Gay*Delta_UK1-epsilon; -Gay*Delta_UK1-epsilon    10*6
    b_cons_coeff1=[Ay_SoftBound;Ay_SoftBound];% 10*1
    % % 将方向盘转角约束和侧向加速度软约束合到一起
    A_cons = [A_cons0;A_cons1]; %20*6
    b_cons_coeff = [b_cons_coeff0;b_cons_coeff1]; %20*1
    Delta_UK1 = kron(ones(Nc,1), FrontWheel_AngleK1_rad);%上一帧的前轮转角
    b_cons = b_cons_coeff+[-Delta_UK1;Delta_UK1;-Gay*eye(Nu*Nc)*Delta_UK1;Gay*eye(Nu*Nc)*Delta_UK1]; %20*1
    
    % % 限值约束,方向盘转角速度上下限,松弛因子epsilon上下限
    mu = single(0.75);
    g = single(9.8);
    dDelta_bound = Du_Max*Ts/single(57.3);% max_steer_rate转角速度限制 0.0082rad = 0.47deg(此处为车轮转角增加，应该转换成方向盘的转角增量)
    dDelta_Bound=kron(ones(Nc,1),dDelta_bound);%5*1
    lb = [-dDelta_Bound;0]; %6*1
    ub = [dDelta_Bound;mu*g-Ay_softbound];%6*1
    % ub = [dDelta_Bound;5*mu*g-Ay_softbound];
    % 边界约束转不等式约束
    [lb_row,~] = size(lb);
    A_cons = [A_cons;eye(lb_row);-eye(lb_row)];
    b_cons = [b_cons;ub;-lb];
    %--------------------------------------------------------------------%
    err = [lateral_error,lateral_error_rate,heading_error,heading_error_rate,FrontWheel_AngleK1_rad]';
    psid_ref = ref_curvature*Veh_Speed;
    
    % 转换后的优化目标函数矩阵
    Row = SoftConstWeight;
    H=[Bt'*Qt*Bt+Rt,zeros(Nu*Nc,1);zeros(1,Nu*Nc),Row]; % Row 
    F=[Bt'*Qt*(At*err+Ct*psid_ref);0];
    %-------------------QP问题求解------------------------%
    % min(J) = 0.5x'Hx + f'x  
    % A_Const*x <= b
    uDelta = MPC_Solver_QPhild(H,F,A_cons,b_cons);% 增加了软约束的变量
    
    FrontWheel_Angle = FrontWheel_AngleK1_rad +uDelta(1); % 取第一个值作为输入
    %--------------前转角反算方向盘转角+弧度转角度---------------------%
    if (FrontWheel_Angle>=0)
        steer_transmission_ratio = veh_params.left_steer_ratio;
    else
        steer_transmission_ratio = veh_params.right_steer_ratio;
    end
    Final_steer_angle_cmd = FrontWheel_Angle * single(57.3) * steer_transmission_ratio; 
    % 反算方向盘转角并转换为角度制deg,输出算法计算角度作为观测，下一步会补偿转向不足。
    steer_angle_cmd = Final_steer_angle_cmd + single(CurrentSteerAngleOffset); % 后期会补充转向不足
    
else
    steer_angle_cmd = SteerAngle;
    Final_steer_angle_cmd = single(0);
    LatError_contribution = single(0);
    LatErrorRate_contribution = single(0);
    HeadingError_contribution = single(0);
    HeadingErrorRate_contribution = single(0);
end
end
function eta = MPC_Solver_QPhild(H,f,A_Const,b)
% 二次规划
% 该算法是原始对偶算法，该方法充分的剖析了优化问题的结构，是求解二次规划问题的一个较好的算法。
% J = 0.5x'Hx + f'x = min
% A_Const*x <= b
[n1,~] = size(A_Const);
eta = -H\f;
kk = single(0);
for i = 1:n1
    if(A_Const(i,:)*eta>b(i))
        kk = kk+single(1);
    else
        kk = kk+single(0);
    end
end
if kk == 0
    return;
end
P = A_Const*(H\A_Const');
d = (A_Const*(H\f)+b);
[n,m] = size(d);
x_ini = zeros(n,m);
lambda = x_ini;
for km = 1:38
    lambda_p = lambda;
    for i = 1:n
        w = P(i,:)*lambda - P(i,i)*lambda(i,1);
        w = w + d(i,1);
        la = -w/P(i,i);
        lambda(i,1) = max(0,la);
    end
    al = (lambda - lambda_p)'*(lambda - lambda_p);
    if(al<10e-8)
        break
    end
end
eta = -H\f -H\A_Const'*lambda;
end
